simulink model "single_in_state_out_free"  (R2021b)
settings: Solver=VariableStepAuto  StartTime=0.0  StopTime=10.0  RelTol=1e-3
settings Model: Creator=den  LastModifiedBy=den

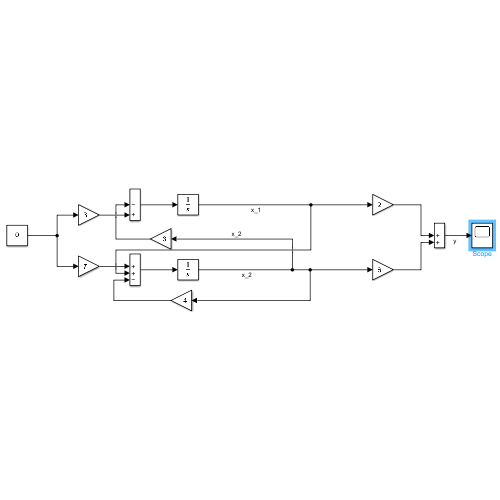
[thumbnail: Simulink's stored preview of the top-level diagram]
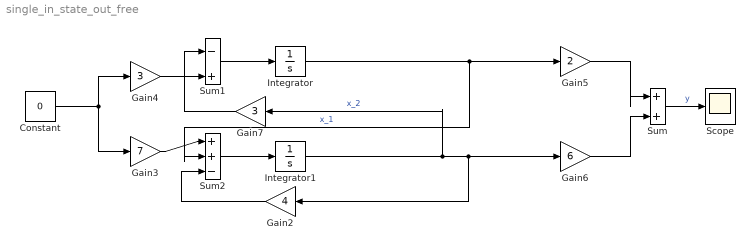
== system single_in_state_out_free ==
  Constant : Constant  Value=0
  Gain2 : Gain  Gain=4
  Gain3 : Gain  Gain=7
  Gain4 : Gain  Gain=3
  Gain5 : Gain  Gain=2
  Gain6 : Gain  Gain=6
  Gain7 : Gain  Gain=3
  Integrator : Integrator  InitialCondition=1
  Integrator1 : Integrator  InitialCondition=0.6
  Scope : Scope
  Sum : Sum  Inputs=|++
  Sum1 : Sum  Inputs=|-+
  Sum2 : Sum  Inputs=|++-
  wires:
  Sum/1 -> Scope/1  "y"
  Gain5/1 -> Sum/1
  Gain6/1 -> Sum/2
  Constant/1 -> Gain3/1, Gain4/1
  Sum1/1 -> Integrator/1
  Sum2/1 -> Integrator1/1
  Integrator/1 -> Sum2/2, Gain5/1  "x_1"
  Integrator1/1 -> Gain6/1, Gain2/1, Gain7/1  "x_2"
  Gain2/1 -> Sum2/3
  Gain3/1 -> Sum2/1
  Gain4/1 -> Sum1/2
  Gain7/1 -> Sum1/1
